simulink model "Plant_model"  (R2020b)
settings: Solver=VariableStepAuto  StartTime=0.0  StopTime=10.0  RelTol=1e-3
settings Model: Creator=hp  LastModifiedBy=hp
settings DataIOCC: SaveOutput=off  SaveTime=off

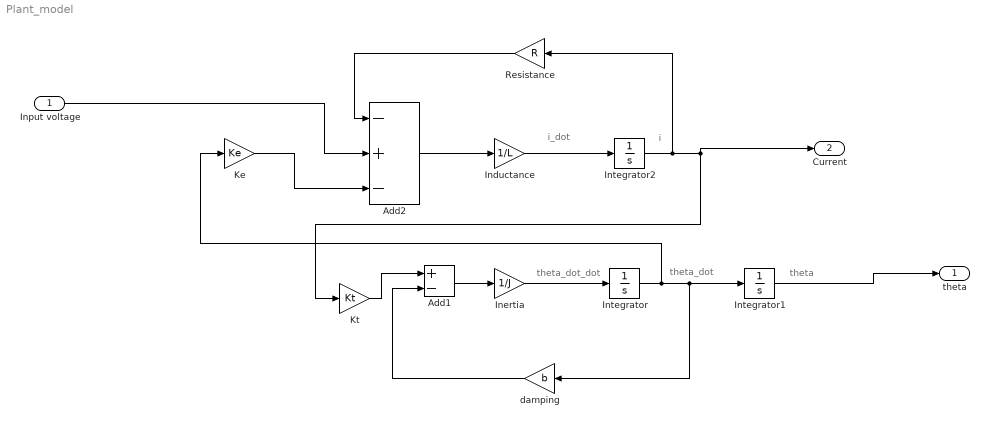
== system Plant_model ==
  note: i
  note: theta_dot_dot
  note: i_dot
  note: theta_dot
  note: theta
  Input voltage : Inport  OutDataTypeStr=double  PortDimensions=1  SampleTime=0
  Add1 : Sum  Inputs=+-
  Add2 : Sum  Inputs=-+-
  Inductance : Gain  Gain=1/L  mask{L=2.75*10^(-6)}
  Inertia : Gain  Gain=1/J  mask{J=3.22*10^(-6)}
  Integrator : Integrator
  Integrator1 : Integrator
  Integrator2 : Integrator
  Ke : Gain  Gain=Ke  mask{Ke=0.0274}
  Kt : Gain  Gain=Kt  mask{Kt=0.0274}
  Resistance : Gain  Gain=R  mask{R=4}
  damping : Gain  Gain=b  mask{b=3.5077*10^(-6)}
  theta : Outport  OutDataTypeStr=double  PortDimensions=1  SampleTime=0
  Current : Outport  Port=2  OutDataTypeStr=double  PortDimensions=1  SampleTime=0
  wires:
  Input voltage/1 -> Add2/2
  damping/1 -> Add1/2
  Ke/1 -> Add2/3
  Integrator/1 -> Ke/1, damping/1, Integrator1/1
  Resistance/1 -> Add2/1
  Add2/1 -> Inductance/1
  Inertia/1 -> Integrator/1
  Integrator2/1 -> Kt/1, Current/1, Resistance/1
  Kt/1 -> Add1/1
  Integrator1/1 -> theta/1
  Inductance/1 -> Integrator2/1
  Add1/1 -> Inertia/1
